simulink model "TwoWheelNeuro"  (R2024b)
settings: Solver=VariableStepAuto  StartTime=0.0  StopTime=2.2  RelTol=1e-3
libraries: neural x1
settings Model: Creator=Dr.Red  LastModifiedBy=Dr.Red

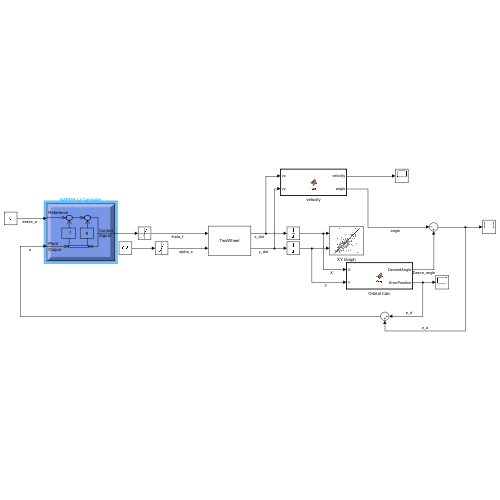
[thumbnail: Simulink's stored preview of the top-level diagram]
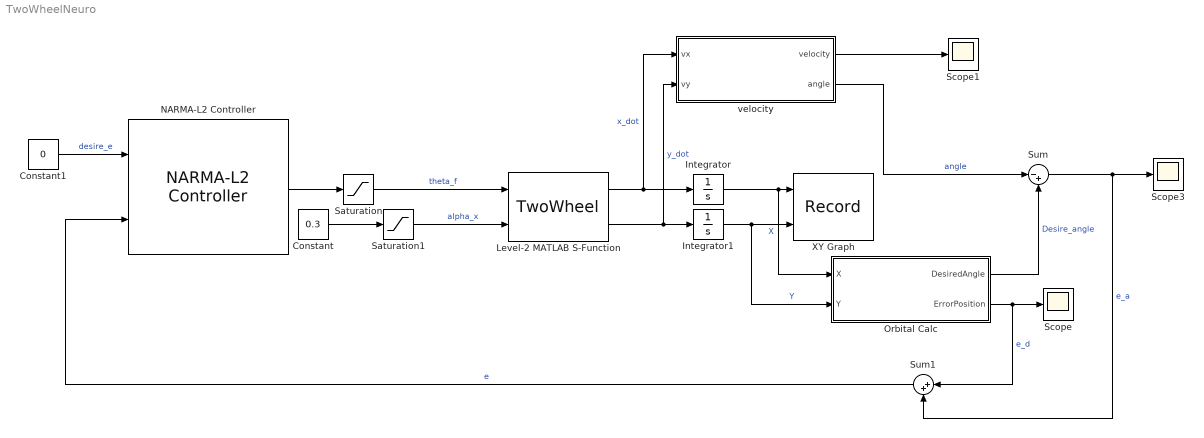
== system TwoWheelNeuro ==
  Constant : Constant  Value=0.3
  Constant1 : Constant  Value=0
  Integrator : Integrator
  Integrator1 : Integrator
  Level-2 MATLAB S-Function : M-S-Function  FunctionName=TwoWheel  Parameters=10,0,0,0
  NARMA-L2 Controller : neural/Control Systems/NARMA-L2 Controller  Normalize=1  IW1_1=[1.6051197891857833522 -4.3203870043674115209;-2.6662633884578776922 4.1091151891405992558;4.1468681384298911041 -2.943051152101508805;-0.012907531436157616833 -4.8304593721178807897;3.8430994564193707852 3.2774582082797087956;-1.2364832546032720195 5.0458657425966464416;5.1091585769244680648 0.49370769415759041543;-1.3359506108825534021 -4.6686033045701584854;3.4423546655225045754 -3.633762278024593062;3.3157790011208057024 -3.9854934586977992517;3.7854982096236868827 -0.061346072205331295124;-4.0238312052470988078 0.11024759032365530342;3.6664109785860232726 3.1238132149945521121]  IW3_2=[3.6948033263158133188 3.4557659626809313913;4.2268193276052912211 2.786224880919671687;-0.10761375657219611479 -5.0313516480608084791;-4.735715209127775438 1.800094253752722917;-1.9754489903210661339 -4.6356008505787684726;4.9649419410896014071 -0.94907446302229092616;3.8934207875154913658 3.2058240903954282608;4.9418711574478519921 0.80613597395582492489;3.7421132418796254626 -3.239937558345860058;3.3673584387036252785 -3.8589026785190334579;2.1651555008582512585 4.5321727660996984355;-4.4788708589031918095 2.5535749256837529941;-2.147512119854346313 4.601323224583036442]  IW5_3=0.90715439344815551603  LW2_1=[1.1707491108004668412 -0.3144770519639901174 1.3389803991800779404 -0.030982281980360362739 0.0016241681370364399739 -0.071230314190635371507 0.30736018033232520574 -0.087152610602200558665 -0.32299262930035693708 0.2849272970329386756 1.459296594140666814 -1.3266634471556681962 0.044399343972538078684]  LW4_3=[0.31758883218058442388 0.60203650396948815704 -0.47926189390362700093 0.20405399475055502334 -0.045130615503027243784 -0.71993997289799083195 0.72579197988840993272 -0.42017963524497187189 -0.41902784832288697547 0.66440378830071722405 -0.63065922527865891922 0.45167035799896676496 -0.66889685370951490473]  LW5_4=0.59791203613559884555  LW6_5=0.0023319441671211839362  LW6_2=0.16575676803781852486  B1=[-5.8455094605270003782;4.5962910818065640939;-3.393349055626437849;2.7840518751750442661;-1.9281388759550148748;0.55609242098327826831;-0.13103820955471182086;-1.5166107992246622427;2.0599007511670581749;2.0469584955930839598;1.8188660781888676965;-3.643004515504967511;5.0484770645367040842]  B2=-0.99934741888996037051  B3=[-5.0429552293888848524;-4.2009984321713780275;3.3941375845695507252;2.5120407009744338822;1.6947332960528846968;-0.7548392106491718101;0.017191302842459909445;1.0155490975856262814;1.7670513050716272208;2.3965035986118108369;3.4375890998342772953;-4.1343701002720658622;-5.0568607559091915959]  B4=-0.74619889126878446994  Limit_output=0  min_output=-Inf  max_output=Inf  Use_Previous_Weights=1  Ts=0.001  S1=13  Ni=2  Nj=1  sim_file=ModelRed  trainfun=trainlm  Use_validation=1  Use_Testing=1  max_i=0.35  min_i=-0.35  max_i_int=0.01  min_i_int=0.005  sam_training=500  epochs=6  minp=-0.34686429890033398937  maxp=0.34819532953002907405  mint=0  maxt=0.34819532953002907405
  Orbital Calc : MATLAB Function  TreatAsAtomicUnit=on
  Saturation : Saturate  UpperLimit=0.3  LowerLimit=-0.3
  Saturation1 : Saturate  UpperLimit=1.5  LowerLimit=-2
  Scope : Scope
  Scope1 : Scope
  Scope3 : Scope
  Sum : Sum  Inputs=|-+
  Sum1 : Sum  Inputs=|++
  XY Graph : Record  FileSettingsInternal="{\"entries\":[{\"content\":{\"excelSettings\":{\"content\":{},\"type\":\"Streamout.ExcelSettings\"}},\"type\":\"Streamout.FileSettingStorage\",\"uuid\":\"\"}],\"packageUris\":[\"http:\\/\\/schema.mathworks.com\\/mf0\\/streamout_blocks\\/R2020a\"],\"version\":\"1.0\"}"  Layout=[1 1]  SignalsInternal="{\"entries\":[{\"content\":{\"signals\":[{\"content\":{\"blockPath\":[],\"dimensions\":[1],\"domain\":\"\",\"lineColor\":\"#a2142f\",\"plots\":[ 1 ],\"port\":1,\"sid\":[\"\"],\"signalID\":1,\"signalName\":\"X\"},\"type\":\"RecordBlkView.Signal\",\"uuid\":\"\"},{\"content\":{\"blockPath\":[],\"dimensions\":[1],\"domain\":\"\",\"lineColor\":\"#139fff\",\"plots\":[ 1 ],\"port\":2,\"sid\":[\"\"],\"signalID\":2,\"signalName\":\"Y\"},\"type\":\"RecordBlkView.Signal\",\"uuid\":\"\"}]},\"type\":\"RecordBlkView.InputSignals\",\"uuid\":\"\"}],\"packageUris\":[\"http:\\/\\/schema.mathworks.com\\/mf0\\/streamout_blocks\\/R2020a\"],\"version\":\"1.0\"}"  VisualizationBindings="{\"xyplotplugin\":{\"info\":[{\"series\":[{\"bindingParametersList\":[{\"parameter\":\"X-Axis\",\"signalID\":1,\"signalName\":\"X\"},{\"parameter\":\"Y-Axis\",\"signalID\":2,\"signalName\":\"Y\"}],\"seriesID\":0}],\"subplotID\":1}]}}"  CompatibilityTag=XY
  velocity : MATLAB Function  TreatAsAtomicUnit=on
  wires:
  Saturation/1 -> Level-2 MATLAB S-Function/1  "theta_f"
  Integrator/1 -> Orbital Calc/1(X), XY Graph/1  "X"
  velocity/1(velocity) -> Scope1/1
  Constant/1 -> Saturation1/1
  Orbital Calc/2(ErrorPosition) -> Sum1/1, Scope/1  "e_d"
  Saturation1/1 -> Level-2 MATLAB S-Function/2  "alpha_x"
  Level-2 MATLAB S-Function/2 -> velocity/2(vy), Integrator1/1  "y_dot"
  Level-2 MATLAB S-Function/1 -> velocity/1(vx), Integrator/1  "x_dot"
  Integrator1/1 -> XY Graph/2, Orbital Calc/2(Y)  "Y"
  velocity/2(angle) -> Sum/1  "angle"
  Orbital Calc/1(DesiredAngle) -> Sum/2  "Desire_angle"
  Constant1/1 -> NARMA-L2 Controller/1  "desire_e"
  Sum/1 -> Scope3/1, Sum1/2  "e_a"
  Sum1/1 -> NARMA-L2 Controller/2  "e"
  NARMA-L2 Controller/1 -> Saturation/1

== matlab function TwoWheelNeuro/Orbital Calc ==
  data: DesiredAngle output; X input; ErrorPosition output; Y input
function [DesiredAngle,ErrorPosition] = fcn(X,Y)
    
    RoundPosition = [0,15];

    Radius = 15;

ErrorPosition = - Radius + power((RoundPosition(1)-X)^2+(RoundPosition(2)-Y)^2,0.5);

DesiredAngle = atan2(X-RoundPosition(1),RoundPosition(2)-Y);

== matlab function TwoWheelNeuro/velocity ==
  data: vx input; velocity output; vy input; angle output
function [velocity,angle] = fcn(vx,vy)
    

velocity = power(vx^2+vy^2,0.5);

angle = atan2(vy,vx);
